simulink model "test"  (R2021b)
settings: Solver=VariableStepAuto  StartTime=0.0  StopTime=10.0  RelTol=1e-3
settings Model: Creator=bearhero  LastModifiedBy=bearhero

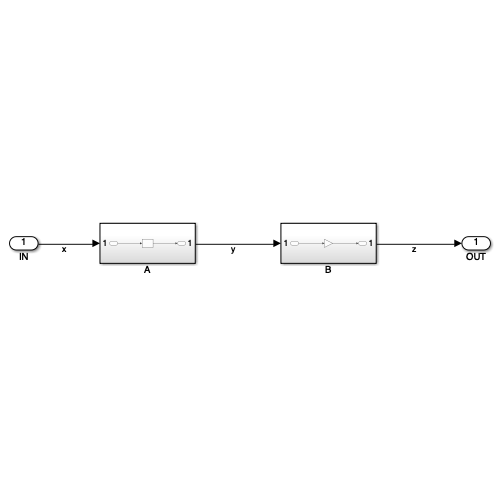
[thumbnail: Simulink's stored preview of the top-level diagram]
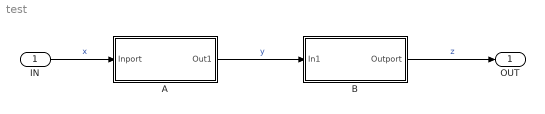
== system test ==
  IN : Inport
  A : Subsystem
  B : Subsystem
  OUT : Outport
  wires:
  IN/1 -> A/1(Inport)  "x"
  A/1(Out1) -> B/1(In1)  "y"
  B/1(Outport) -> OUT/1  "z"

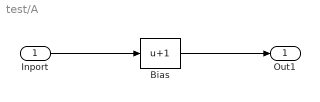
== system test/A ==
  Inport : Inport
  Bias : Bias  Bias=1
  Out1 : Outport
  wires:
  Inport/1 -> Bias/1
  Bias/1 -> Out1/1

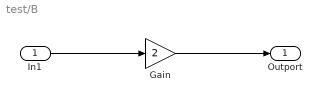
== system test/B ==
  In1 : Inport
  Gain : Gain  Gain=2
  Outport : Outport
  wires:
  In1/1 -> Gain/1
  Gain/1 -> Outport/1
